simulink model "simulink_model_a"  (R2018b)
settings: Solver=VariableStepAuto  StartTime=0.0  StopTime=100  RelTol=1e-3
libraries: fuzblock x1
settings Model: Creator=XAVIER  LastModifiedBy=jorge

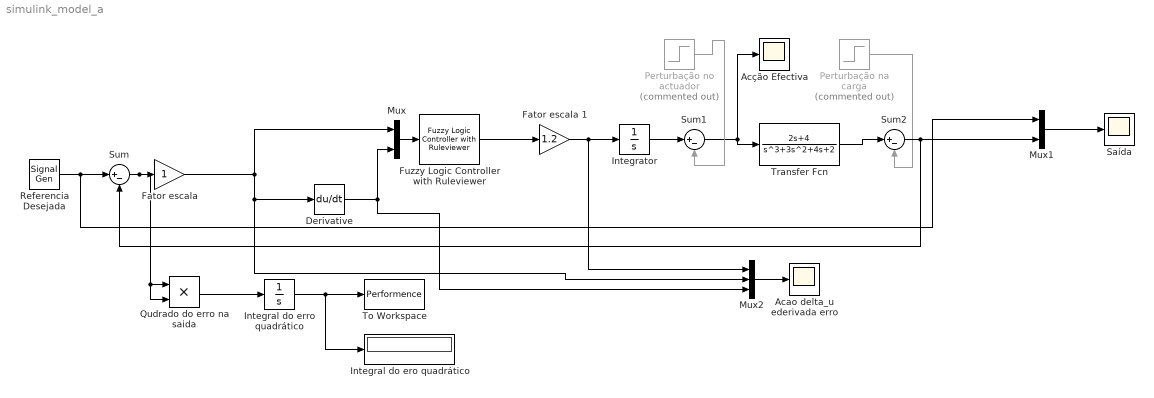
== system simulink_model_a ==
  "Acao delta_u ederivada erro " : Scope
  Acção Efectiva : Scope
  Derivative : Derivative
  "Fator escala " : Gain
  Fator escala 1 : Gain  Gain=1.2
  Fuzzy Logic Controller with Ruleviewer : fuzblock/Fuzzy Logic  Controller  with Ruleviewer  fismatrix=mycontroler  Ts=2
  "Integral do ero quadrático " : Display
  Integral do erro quadrático : Integrator
  Integrator : Integrator
  Mux : Mux  Inputs=2
  Mux1 : Mux  Inputs=2
  Mux2 : Mux  Inputs=3
  "Perturbação na carga " : Step  Commented=on  Time=225  SampleTime=1
  "Perturbação no actuador " : Step  Commented=on  Time=150  SampleTime=1
  "Qudrado do erro na saida " : Product
  Referencia Desejada : SignalGenerator  WaveForm=square  Frequency=0.009
  Saída : Scope
  Sum : Sum  Inputs=|+-
  Sum1 : Sum  Inputs=|+-
  Sum2 : Sum  Inputs=|+-
  To Workspace : ToWorkspace  VariableName=Performence  SaveFormat=Timeseries  SampleTime=-1
  Transfer Fcn : TransferFcn  Numerator=[2 4]  Denominator=[1 3 4 2]
  wires:
  Integral do erro quadrático/1 -> "Integral do ero quadrático "/1, To Workspace/1
  Mux1/1 -> Saída/1
  Mux2/1 -> "Acao delta_u ederivada erro "/1
  "Perturbação na carga "/1 -> Sum2/2
  Sum2/1 -> Sum/2, Mux1/2
  Fator escala 1/1 -> Mux2/1, Integrator/1
  Derivative/1 -> Mux2/3, Mux/2
  Sum1/1 -> Acção Efectiva/1, Transfer Fcn/1
  "Qudrado do erro na saida "/1 -> Integral do erro quadrático/1
  Mux/1 -> Fuzzy Logic Controller with Ruleviewer/1
  Transfer Fcn/1 -> Sum2/1
  "Perturbação no actuador "/1 -> Sum1/2
  Referencia Desejada/1 -> Mux1/1, Sum/1
  "Fator escala "/1 -> Mux/1, Mux2/2, Derivative/1
  Sum/1 -> "Qudrado do erro na saida "/2, "Qudrado do erro na saida "/1, "Fator escala "/1
  Integrator/1 -> Sum1/1
  Fuzzy Logic Controller with Ruleviewer/1 -> Fator escala 1/1
